simulink model "Simulation"  (R2018a)
settings: Solver=VariableStepAuto  StartTime=0.0  StopTime=10.0  RelTol=1e-3
libraries: simulink_extras x1
settings Model: Creator=chrros005  LastModifiedBy=chrros005

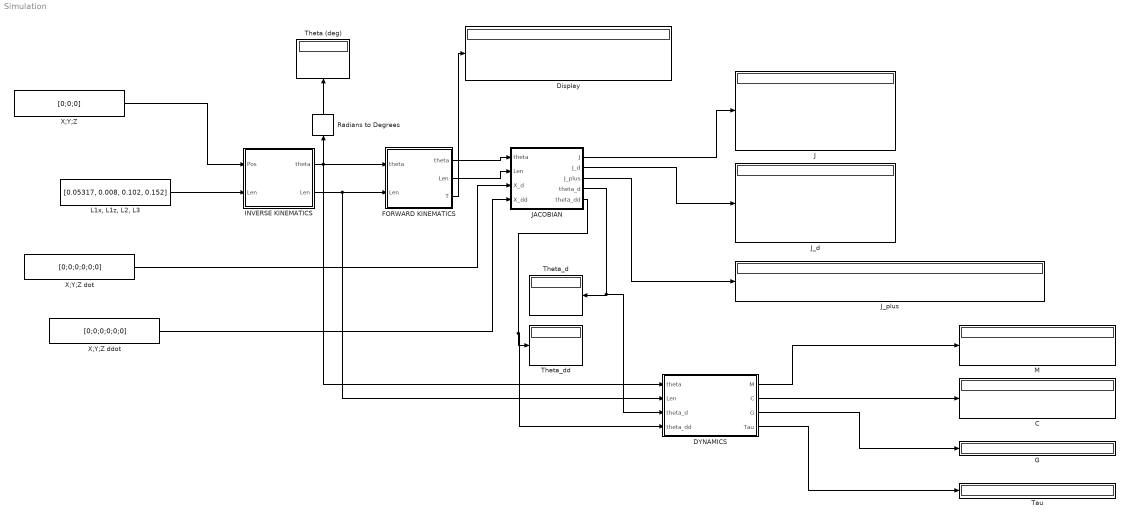
== system Simulation ==
  C : Display
  "DYNAMICS " : MATLAB Function  TreatAsAtomicUnit=on
  Display : Display
  "FORWARD KINEMATICS " : MATLAB Function  TreatAsAtomicUnit=on
  G : Display
  "INVERSE KINEMATICS " : MATLAB Function  TreatAsAtomicUnit=on
  J : Display
  JACOBIAN : MATLAB Function  TreatAsAtomicUnit=on
  J_d : Display
  "J_plus " : Display
  "L1x, L1z, L2, L3" : Constant  Value=[0.05317, 0.008, 0.102, 0.152]
  M : Display
  Radians to Degrees : simulink_extras/Transformations/Radians to Degrees
  Tau : Display
  Theta (deg) : Display
  Theta_d : Display
  Theta_dd : Display
  "X;Y;Z " : Constant  Value=[0;0;0]
  X;Y;Z ddot : Constant  Value=[0;0;0;0;0;0]
  X;Y;Z dot : Constant  Value=[0;0;0;0;0;0]
  wires:
  "X;Y;Z "/1 -> "INVERSE KINEMATICS "/1(Pos)
  "L1x, L1z, L2, L3"/1 -> "INVERSE KINEMATICS "/2("Len ")
  "INVERSE KINEMATICS "/1(theta) -> "FORWARD KINEMATICS "/1("theta "), "DYNAMICS "/1(theta), Radians to Degrees/1
  "INVERSE KINEMATICS "/2(Len) -> "DYNAMICS "/2(Len), "FORWARD KINEMATICS "/2("Len ")
  "FORWARD KINEMATICS "/1(theta) -> JACOBIAN/1(theta)
  "FORWARD KINEMATICS "/2(Len) -> JACOBIAN/2(Len)
  JACOBIAN/1(J) -> J/1
  JACOBIAN/2(J_d) -> J_d/1
  JACOBIAN/3(J_plus) -> "J_plus "/1
  X;Y;Z dot/1 -> JACOBIAN/3(X_d)
  JACOBIAN/4(theta_d) -> "DYNAMICS "/3(theta_d), Theta_d/1
  JACOBIAN/5(theta_dd) -> "DYNAMICS "/4(theta_dd), Theta_dd/1
  X;Y;Z ddot/1 -> JACOBIAN/4(X_dd)
  Radians to Degrees/1 -> Theta (deg)/1
  "DYNAMICS "/1(M) -> M/1
  "DYNAMICS "/2(C) -> C/1
  "DYNAMICS "/3(G) -> G/1
  "DYNAMICS "/4(Tau) -> Tau/1
  "FORWARD KINEMATICS "/3(T) -> Display/1

== matlab function Simulation/FORWARD KINEMATICS  ==
  data: theta output; Len output; theta input; T output; Len input
function [theta,Len,T]= FWD(theta, Len)
    
    
    theta1 = theta(1);
    theta2 = theta(2);
    theta3 = theta(3);
   
    L1x = Len(1);
    L1z = Len(2);
    L2 = Len(3);
    L3 = Len(4); 
    


  
    T = [ cos(theta2 + theta3)*cos(theta1), -sin(theta1), -sin(theta2 + theta3)*cos(theta1), cos(theta1)*(L1x + L3*cos(theta2 + theta3) + L2*cos(theta2));
          cos(theta2 + theta3)*sin(theta1),  cos(theta1), -sin(theta2 + theta3)*sin(theta1), sin(theta1)*(L1x + L3*cos(theta2 + theta3) + L2*cos(theta2));
                      sin(theta2 + theta3),            0,              cos(theta2 + theta3),               L1z + L3*sin(theta2 + theta3) + L2*sin(theta2);
                                         0,            0,                                 0,                                                            1];

== matlab function Simulation/INVERSE KINEMATICS  ==
  data: Pos input; theta output; Len input; Len output
function [theta, Len]= INV(Pos,Len)

    x = Pos(1);
    y = Pos(2);
    z = Pos(3);
    
    L1x = Len(1);
    L1z = Len(2);
    L2 = Len(3);
    L3 = Len(4);
    
    theta1 =  ( atan2(y,x) );
    
    C3 = ( ( x - L1x*cos(theta1) )^2 + ( y - L1x*sin(theta1) )^2 + ( z - L1z )^2 - L2^2 - L3^2 )/( 2*L2*L3 );
    S3 = -sqrt(1 - C3^2);

    theta2 =  ( atan2( z-L1z, sqrt( (x-L1x*cos(theta1))^2 + (y - L1x*sin(theta1))^2 ) ) - atan2(L3*S3, L2 + L3*C3) );

    theta3 =  ( atan2(S3, C3) );
    
    theta = [theta1; theta2; theta3];

== matlab function Simulation/JACOBIAN ==
  data: theta input; Len input; X_d input; J output; J_d output; J_plus output; theta_d output; theta_dd output; X_dd input
function [J, J_d, J_plus, theta_d, theta_dd]= JAC(theta, Len, X_d, X_dd)

    theta1 = theta(1);
    theta2 = theta(2);
    theta3 = theta(3);
    
    L1x = Len(1);
    L1z = Len(2);
    L2 = Len(3);
    L3 = Len(4);
   
    J = [-sin(theta1)*(L1x + L3*cos(theta2 + theta3) + L2*cos(theta2)), cos(theta1)*(L3*sin(theta2 + theta3) + L2*sin(theta2)), L3*sin(theta2 + theta3)*cos(theta1);
        cos(theta1)*(L1x + L3*cos(theta2 + theta3) + L2*cos(theta2)), sin(theta1)*(L3*sin(theta2 + theta3) + L2*sin(theta2)), L3*sin(theta2 + theta3)*sin(theta1);
                                                             0,             - L3*cos(theta2 + theta3) - L2*cos(theta2),            -L3*cos(theta2 + theta3);
                                                             0,                                           -sin(theta1),                        -sin(theta1);
                                                             0,                                            cos(theta1),                         cos(theta1);
                                                             1,                                                      0,                                   0]
                                                        
    J_plus = [ -(2*sin(theta1)*(L1x + L3*cos(theta2 + theta3) + L2*cos(theta2)))/(L2^2*cos(2*theta2) + L3^2*cos(2*theta2 + 2*theta3) + L2^2 + L3^2 + 2*L1x^2 + 2*L2*L3*cos(2*theta2 + theta3) + 4*L3*L1x*cos(theta2 + theta3) + 2*L2*L3*cos(theta3) + 4*L2*L1x*cos(theta2) + 2), (2*cos(theta1)*(L1x + L3*cos(theta2 + theta3) + L2*cos(theta2)))/(L2^2*cos(2*theta2) + L3^2*cos(2*theta2 + 2*theta3) + L2^2 + L3^2 + 2*L1x^2 + 2*L2*L3*cos(2*theta2 + theta3) + 4*L3*L1x*cos(theta2 + theta3) + 2*L2*L3*cos(theta3) + 4*L2*L1x*cos(theta2) + 2),                                                                                                                                                                                 0,                                                                         0,                                                                        0, 1/((L2^2*cos(2*theta2))/2 + (L3^2*cos(2*theta2 + 2*theta3))/2 + L2^2/2 + L3^2/2 + L1x^2 + L2*L3*cos(2*theta2 + theta3) + 2*L3*L1x*cos(theta2 + theta3) + L2*L3*cos(theta3) + 2*L2*L1x*cos(theta2) + 1);
                                                                                                                                                     (cos(theta1)*(sin(theta2) - (L3^2*sin(theta2 + 2*theta3))/2 + (L3^2*sin(theta2))/2))/(L2*(L3^2 - L3^2*cos(theta3)^2 + 1)),                                                                                                                                       (sin(theta1)*(sin(theta2) - (L3^2*sin(theta2 + 2*theta3))/2 + (L3^2*sin(theta2))/2))/(L2*(L3^2 - L3^2*cos(theta3)^2 + 1)),                                                                            -(2*cos(theta2) - L3^2*cos(theta2 + 2*theta3) + L3^2*cos(theta2))/(L2*(L3^2 - L3^2*cos(2*theta3) + 2)),         (L3*cos(theta3)*sin(theta1))/(L2*(L3^2 - L3^2*cos(theta3)^2 + 1)),       -(L3*cos(theta1)*cos(theta3))/(L2*(L3^2 - L3^2*cos(theta3)^2 + 1)),                                                                                                                                                                                                      0;
                                                                               (cos(theta1)*(L3^2*cos(theta3)^2*sin(theta2) - L3^2*sin(theta2) - sin(theta2) + L3^2*cos(theta2)*cos(theta3)*sin(theta3) + L2*L3*cos(theta2)*sin(theta3)))/(L2*(L3^2 - L3^2*cos(theta3)^2 + 1)),                                                                 (sin(theta1)*(L3^2*cos(theta3)^2*sin(theta2) - L3^2*sin(theta2) - sin(theta2) + L3^2*cos(theta2)*cos(theta3)*sin(theta3) + L2*L3*cos(theta2)*sin(theta3)))/(L2*(L3^2 - L3^2*cos(theta3)^2 + 1)), (cos(theta2) + L3^2*cos(theta2) - L3^2*cos(theta2)*cos(theta3)^2 + L3^2*cos(theta3)*sin(theta2)*sin(theta3) + L2*L3*sin(theta2)*sin(theta3))/(L2*(L3^2 - L3^2*cos(theta3)^2 + 1)), -(sin(theta1)*(L2 + L3*cos(theta3)))/(L2*(L3^2 - L3^2*cos(theta3)^2 + 1)), (cos(theta1)*(L2 + L3*cos(theta3)))/(L2*(L3^2 - L3^2*cos(theta3)^2 + 1)),                                                                                                                                                                                                      0];
 
 
   
    theta_d =  J_plus*X_d; 
    theta1_d = theta_d(1);
    theta2_d = theta_d(2);
    theta3_d = theta_d(3);
                                                            

    J_d =   [   theta2_d*sin(theta1)*(L3*sin(theta2 + theta3) + L2*sin(theta2)) - theta1_d*cos(theta1)*(L1x + L3*cos(theta2 + theta3) + L2*cos(theta2)) + L3*theta3_d*sin(theta2 + theta3)*sin(theta1), theta2_d*cos(theta1)*(L3*cos(theta2 + theta3) + L2*cos(theta2)) - theta1_d*sin(theta1)*(L3*sin(theta2 + theta3) + L2*sin(theta2)) + L3*theta3_d*cos(theta2 + theta3)*cos(theta1), L3*theta2_d*cos(theta2 + theta3)*cos(theta1) + L3*theta3_d*cos(theta2 + theta3)*cos(theta1) - L3*theta1_d*sin(theta2 + theta3)*sin(theta1);
             - theta2_d*cos(theta1)*(L3*sin(theta2 + theta3) + L2*sin(theta2)) - theta1_d*sin(theta1)*(L1x + L3*cos(theta2 + theta3) + L2*cos(theta2)) - L3*theta3_d*sin(theta2 + theta3)*cos(theta1), theta1_d*cos(theta1)*(L3*sin(theta2 + theta3) + L2*sin(theta2)) + theta2_d*sin(theta1)*(L3*cos(theta2 + theta3) + L2*cos(theta2)) + L3*theta3_d*cos(theta2 + theta3)*sin(theta1), L3*theta1_d*sin(theta2 + theta3)*cos(theta1) + L3*theta2_d*cos(theta2 + theta3)*sin(theta1) + L3*theta3_d*cos(theta2 + theta3)*sin(theta1);
                                                                                                                                                                                                    0,                                                                                           theta2_d*(L3*sin(theta2 + theta3) + L2*sin(theta2)) + L3*theta3_d*sin(theta2 + theta3),                                                                        L3*theta2_d*sin(theta2 + theta3) + L3*theta3_d*sin(theta2 + theta3);
                                                                                                                                                                                                    0,                                                                                                                                                            -theta1_d*cos(theta1),                                                                                                                      -theta1_d*cos(theta1);
                                                                                                                                                                                                    0,                                                                                                                                                            -theta1_d*sin(theta1),                                                                                                                      -theta1_d*sin(theta1);
                                                                                                                                                                                                    0,                                                                                                                                                                                0,                                                                                                                                          0];
    theta_dd = J_plus*( X_dd - J_d*theta_d );

== matlab function Simulation/DYNAMICS  ==
  data: theta input; Len input; M output; C output; G output; Tau output; theta_d input; theta_dd input
function [M,C,G,Tau]= DYN(theta, Len, theta_d,theta_dd)

    L1x = Len(1);
    L1z = Len(2);
    L2 = Len(3);
    L3 = Len(4)

    theta1 = theta(1);
    theta2 = theta(2);
    theta3 = theta(3);
    
    theta1_d= theta_d(1);
    theta2_d= theta_d(2);
    theta3_d= theta_d(3);
    
    L1xc = L1x/2;
    L1zc = L1z/2;
    L2c = L2/2;
    L3c = L3/2;
    
    m = [0.14327;0.04977;0.15456];
    m1 = m(1);
    m2 = m(2);
    m3 = m(3);
    g = 9.80655               
                 
    M = [ (L2c^2*m2)/2 + (L2c^2*m3)/2 + (L3c^2*m3)/2 + L1xc^2*m1 + L1xc^2*m2 + L1xc^2*m3 + (L2c^2*m2*cos(2*theta2))/2 + (L2c^2*m3*cos(2*theta2))/2 + (L3c^2*m3*cos(2*theta2 + 2*theta3))/2 + 2*L3c*L1xc*m3*cos(theta2 + theta3) + L2c*L3c*m3*cos(theta3) + 2*L2c*L1xc*m2*cos(theta2) + 2*L2c*L1xc*m3*cos(theta2) + L2c*L3c*m3*cos(2*theta2 + theta3) + 36456699500413941/36893488147419103232,                                                         0,                              0;
                                                                                                                                                                                                                                                                                                                                                                                           0, L2c^2*m2 + L2c^2*m3 + L3c^2*m3 + 2*L2c*L3c*m3*cos(theta3), L3c*m3*(L3c + L2c*cos(theta3));
                                                                                                                                                                                                                                                                                                                                                                                           0,                            L3c*m3*(L3c + L2c*cos(theta3)),                       L3c^2*m3];
 

    C = [ - theta3_d*((L3c^2*m3*sin(2*theta2 + 2*theta3))/2 + L3c*L1xc*m3*sin(theta2 + theta3) + (L2c*L3c*m3*sin(theta3))/2 + (L2c*L3c*m3*sin(2*theta2 + theta3))/2) - theta2_d*((L2c^2*m2*sin(2*theta2))/2 + (L2c^2*m3*sin(2*theta2))/2 + (L3c^2*m3*sin(2*theta2 + 2*theta3))/2 + L3c*L1xc*m3*sin(theta2 + theta3) + L2c*L1xc*m2*sin(theta2) + L2c*L1xc*m3*sin(theta2) + L2c*L3c*m3*sin(2*theta2 + theta3)), -theta1_d*((L2c^2*m2*sin(2*theta2))/2 + (L2c^2*m3*sin(2*theta2))/2 + (L3c^2*m3*sin(2*theta2 + 2*theta3))/2 + L3c*L1xc*m3*sin(theta2 + theta3) + L2c*L1xc*m2*sin(theta2) + L2c*L1xc*m3*sin(theta2) + L2c*L3c*m3*sin(2*theta2 + theta3)), -theta1_d*((L3c^2*m3*sin(2*theta2 + 2*theta3))/2 + L3c*L1xc*m3*sin(theta2 + theta3) + (L2c*L3c*m3*sin(theta3))/2 + (L2c*L3c*m3*sin(2*theta2 + theta3))/2);
                                                                                                                                                                       theta1_d*((L2c^2*m2*sin(2*theta2))/2 + (L2c^2*m3*sin(2*theta2))/2 + (L3c^2*m3*sin(2*theta2 + 2*theta3))/2 + L3c*L1xc*m3*sin(theta2 + theta3) + L2c*L1xc*m2*sin(theta2) + L2c*L1xc*m3*sin(theta2) + L2c*L3c*m3*sin(2*theta2 + theta3)),                                                                                                                                                                                                       -L2c*L3c*m3*theta3_d*sin(theta3),                                                                                       - L2c*L3c*m3*theta2_d*sin(theta3) - L2c*L3c*m3*theta3_d*sin(theta3);
                                                                                                                                                                                                                                                    theta1_d*((L3c^2*m3*sin(2*theta2 + 2*theta3))/2 + L3c*L1xc*m3*sin(theta2 + theta3) + (L2c*L3c*m3*sin(theta3))/2 + (L2c*L3c*m3*sin(2*theta2 + theta3))/2),                                                                                                                                                                                                        L2c*L3c*m3*theta2_d*sin(theta3),                                                                                                                                                         0];
         
    G = [ L2c*g*m2*cos(theta1);
            g*m3*(L3c*cos(theta2 + theta3) + L2*cos(theta2));
            L3c*g*m3*cos(theta2 + theta3)];
    
        
    Tau = M*theta_dd + C*theta_d + G;
